simulink model "stugverter_hil"  (R2026a)
settings: Solver=VariableStepAuto  StopTime=0.8  MaxStep=1e-5
PreLoadFcn:
  | if exist('init', 'file') ~= 2,   pDir = fileparts(fileparts(which(bdroot)));   if isempty(pDir), pDir = pwd; end;   addpath(fullfile(pDir, 'scripts'));   addpath(fullfile(pDir, 'models'));   addpath(pDir); end; init;
InitFcn:
  | if exist('init', 'file') ~= 2,   pDir = fileparts(fileparts(which(bdroot)));   if isempty(pDir), pDir = pwd; end;   addpath(fullfile(pDir, 'scripts'));   addpath(fullfile(pDir, 'models'));   addpath(pDir); end; init;
undefined symbols (not defined in the file): foc, FOC_20kHz, g_duty_u, g_duty_v, g_duty_w, g_foc_exec_time_us, g_foc_isr_counter, g_hil_adc_curr_u, g_hil_adc_curr_v, g_hil_adc_curr_w, g_hil_adc_res_cos, g_hil_adc_res_sin, g_hil_mode_enable, g_spd_ref_rpm, sensor
libraries: xcpprotocollib x3
settings Model: Creator=niklasprobst  LastModifiedBy=probst
settings DebuggingCC: ParameterPrecisionLossMsg=none

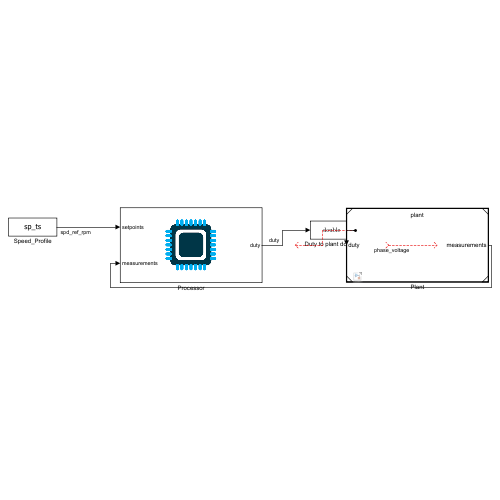
[thumbnail: Simulink's stored preview of the top-level diagram]
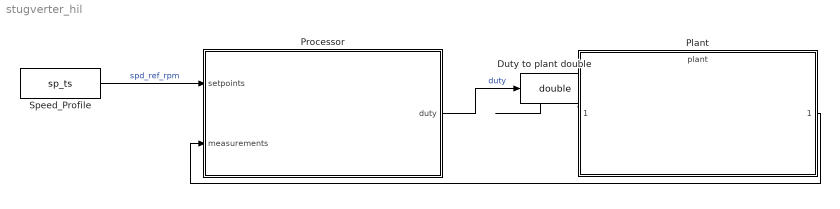
== system stugverter_hil ==
  Duty to plant double : DataTypeConversion  OutDataTypeStr=double  SaturateOnIntegerOverflow=off  RndMeth=Floor
  Plant : ModelReference  ModelNameDialog=plant  SimulationMode=Normal  ModelReferenceVersion=1.2
  Processor : Subsystem
      settings: OpenFcn=open_system(gcb, 'force');
  Speed_Profile : FromWorkspace  VariableName=sp_ts
  wires:
  Speed_Profile/1 -> Processor/1(setpoints)  "spd_ref_rpm"
  ? -> ?  "phase_voltage"
  Processor/1(duty) -> Duty to plant double/1  "duty"
  Duty to plant double/1 -> Plant/1
  Plant/1 -> Processor/2(measurements)

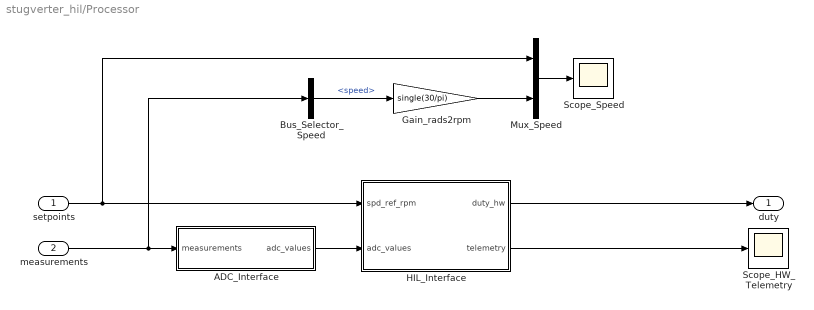
== system stugverter_hil/Processor ==
  setpoints : Inport  OutDataTypeStr=single
  measurements : Inport  Port=2  OutDataTypeStr=Bus: plant_measurement
  ADC_Interface : Subsystem
  Bus_Selector_Speed : BusSelector  OutputSignals=speed
  Gain_rads2rpm : Gain  Gain=single(30/pi)  OutDataTypeStr=single
  HIL_Interface : Subsystem
  Mux_Speed : Mux  Inputs=2
  Scope_HW_Telemetry : Scope
      settings: ActiveDisplayYMinimum=2.3463782313488107E+7  ActiveDisplayYMaximum=2.348257899228869E+7  DataLoggingVariableName=scope_hw_telemetry
  Scope_Speed : Scope
      settings: ActiveDisplayYMinimum=-579.96374511718739  ActiveDisplayYMaximum=5219.6737060546875  DataLoggingVariableName=scope_speed
  duty : Outport
  wires:
  measurements/1 -> ADC_Interface/1(measurements), Bus_Selector_Speed/1
  setpoints/1 -> HIL_Interface/1(spd_ref_rpm), Mux_Speed/1
  ADC_Interface/1(adc_values) -> HIL_Interface/2(adc_values)
  HIL_Interface/1(duty_hw) -> duty/1
  HIL_Interface/2(telemetry) -> Scope_HW_Telemetry/1
  Bus_Selector_Speed/1 -> Gain_rads2rpm/1  "<speed>"
  Gain_rads2rpm/1 -> Mux_Speed/2
  Mux_Speed/1 -> Scope_Speed/1

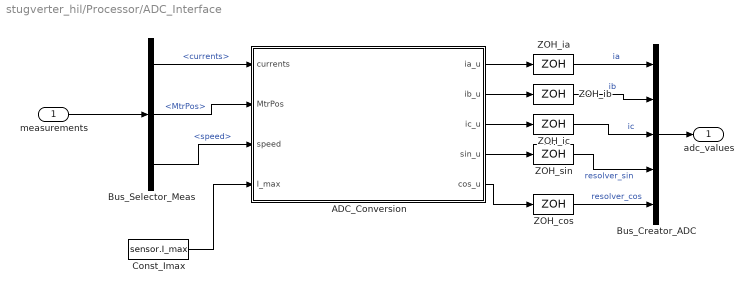
== system stugverter_hil/Processor/ADC_Interface ==
  measurements : Inport  OutDataTypeStr=Bus: plant_measurement
  ADC_Conversion : MATLAB Function  TreatAsAtomicUnit=on
  Bus_Creator_ADC : BusCreator  Inputs=5  OutDataTypeStr=Bus: adc_values  NonVirtualBus=on
  Bus_Selector_Meas : BusSelector  OutputSignals=currents,MtrPos,speed
  Const_Imax : Constant  Value=sensor.I_max
  ZOH_cos : ZeroOrderHold  SampleTime=foc.Ts
  ZOH_ia : ZeroOrderHold  SampleTime=foc.Ts
  ZOH_ib : ZeroOrderHold  SampleTime=foc.Ts
  ZOH_ic : ZeroOrderHold  SampleTime=foc.Ts
  ZOH_sin : ZeroOrderHold  SampleTime=foc.Ts
  adc_values : Outport  OutDataTypeStr=Bus: adc_values
  wires:
  measurements/1 -> Bus_Selector_Meas/1
  Bus_Selector_Meas/1 -> ADC_Conversion/1(currents)  "<currents>"
  Bus_Selector_Meas/2 -> ADC_Conversion/2(MtrPos)  "<MtrPos>"
  ADC_Conversion/1(ia_u) -> ZOH_ia/1
  ZOH_ia/1 -> Bus_Creator_ADC/1  "ia"
  ADC_Conversion/2(ib_u) -> ZOH_ib/1
  ZOH_ib/1 -> Bus_Creator_ADC/2  "ib"
  ADC_Conversion/3(ic_u) -> ZOH_ic/1
  ZOH_ic/1 -> Bus_Creator_ADC/3  "ic"
  ADC_Conversion/4(sin_u) -> ZOH_sin/1
  ZOH_sin/1 -> Bus_Creator_ADC/4  "resolver_sin"
  ADC_Conversion/5(cos_u) -> ZOH_cos/1
  ZOH_cos/1 -> Bus_Creator_ADC/5  "resolver_cos"
  Bus_Creator_ADC/1 -> adc_values/1
  Bus_Selector_Meas/3 -> ADC_Conversion/3(speed)  "<speed>"
  Const_Imax/1 -> ADC_Conversion/4(I_max)

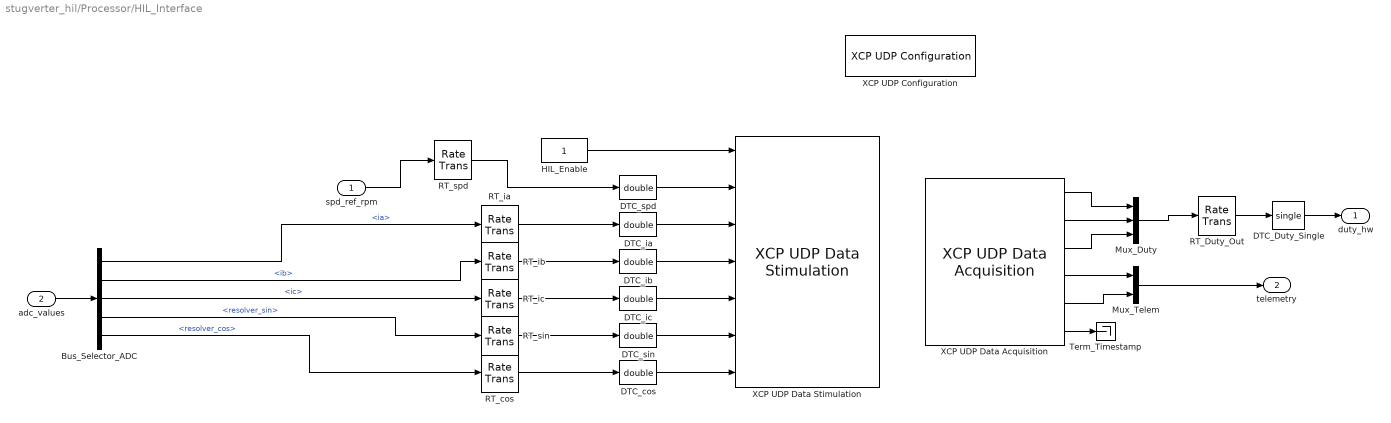
== system stugverter_hil/Processor/HIL_Interface ==
  spd_ref_rpm : Inport
  adc_values : Inport  Port=2
  Bus_Selector_ADC : BusSelector  OutputSignals=ia,ib,ic,resolver_sin,resolver_cos
  DTC_Duty_Single : DataTypeConversion  OutDataTypeStr=single  SaturateOnIntegerOverflow=off  RndMeth=Floor
  DTC_cos : DataTypeConversion  OutDataTypeStr=double  SaturateOnIntegerOverflow=off  RndMeth=Floor
  DTC_ia : DataTypeConversion  OutDataTypeStr=double  SaturateOnIntegerOverflow=off  RndMeth=Floor
  DTC_ib : DataTypeConversion  OutDataTypeStr=double  SaturateOnIntegerOverflow=off  RndMeth=Floor
  DTC_ic : DataTypeConversion  OutDataTypeStr=double  SaturateOnIntegerOverflow=off  RndMeth=Floor
  DTC_sin : DataTypeConversion  OutDataTypeStr=double  SaturateOnIntegerOverflow=off  RndMeth=Floor
  DTC_spd : DataTypeConversion  OutDataTypeStr=double  SaturateOnIntegerOverflow=off  RndMeth=Floor
  HIL_Enable : Constant  OutDataTypeStr=double  SampleTime=foc.Ts
  Mux_Duty : Mux  Inputs=3
  Mux_Telem : Mux  Inputs=2
  RT_Duty_Out : RateTransition  Deterministic=off  InitialCondition=0.5  OutPortSampleTime=foc.Ts
  RT_cos : RateTransition  Deterministic=off  InitialCondition=2048  OutPortSampleTime=foc.Ts
  RT_ia : RateTransition  Deterministic=off  InitialCondition=2048  OutPortSampleTime=foc.Ts
  RT_ib : RateTransition  Deterministic=off  InitialCondition=2048  OutPortSampleTime=foc.Ts
  RT_ic : RateTransition  Deterministic=off  InitialCondition=2048  OutPortSampleTime=foc.Ts
  RT_sin : RateTransition  Deterministic=off  InitialCondition=2048  OutPortSampleTime=foc.Ts
  RT_spd : RateTransition  Deterministic=off  OutPortSampleTime=foc.Ts
  Term_Timestamp : Terminator
  XCP UDP Configuration : xcpprotocollib/UDP/XCP UDP Configuration  Priority=-100  SlaveName=TC387  SlaveID=1  A2LFile=C:\Users\probst\Desktop\stugverter\firmware\stugverter.a2l  EnableSecurity=off  ConnectMode=off  EnableStatus=off  SampleTime=foc.Ts  HeaderErrDet=on  CTRScheme=One counter for all CTOs and DTOs  LocalAddress=192.168.0.100  LocalPort=auto  DAQTimeout=Inf
      settings: LibrarySourceBlock=vntxcplib/UDP/XCP UDP Configuration
  XCP UDP Data Acquisition : xcpprotocollib/UDP/XCP UDP Data Acquisition  SlaveName=TC387  A2LFile=C:\Users\probst\Desktop\stugverter\firmware\stugverter.a2l  EventName=FOC_20kHz (50us)  SelectedMeasurements=g_duty_u;g_duty_v;g_duty_w;g_foc_isr_counter;g_foc_exec_time_us  DAQPriority=0  SampleTime=foc.Ts  EnableTimestamp=on  InputOrOutputDatatype=Raw values as double (no Compu method conversion)
      settings: LibrarySourceBlock=vntxcplib/UDP/XCP UDP Data Acquisition
  XCP UDP Data Stimulation : xcpprotocollib/UDP/XCP UDP Data Stimulation  SlaveName=TC387  A2LFile=C:\Users\probst\Desktop\stugverter\firmware\stugverter.a2l  EventName=FOC_20kHz (50us)  SelectedMeasurements=g_hil_mode_enable;g_spd_ref_rpm;g_hil_adc_curr_u;g_hil_adc_curr_v;g_hil_adc_curr_w;g_hil_adc_res_sin;g_hil_adc_res_cos  EnableTimestamp=off  InputOrOutputDatatype=Raw values as double (no Compu method conversion)
      settings: LibrarySourceBlock=vntxcplib/UDP/XCP UDP Data Stimulation
  duty_hw : Outport
  telemetry : Outport  Port=2
  wires:
  adc_values/1 -> Bus_Selector_ADC/1
  HIL_Enable/1 -> XCP UDP Data Stimulation/1
  DTC_spd/1 -> XCP UDP Data Stimulation/2
  DTC_ia/1 -> XCP UDP Data Stimulation/3
  DTC_ib/1 -> XCP UDP Data Stimulation/4
  DTC_ic/1 -> XCP UDP Data Stimulation/5
  DTC_sin/1 -> XCP UDP Data Stimulation/6
  DTC_cos/1 -> XCP UDP Data Stimulation/7
  XCP UDP Data Acquisition/1 -> Mux_Duty/1
  XCP UDP Data Acquisition/2 -> Mux_Duty/2
  XCP UDP Data Acquisition/3 -> Mux_Duty/3
  DTC_Duty_Single/1 -> duty_hw/1
  XCP UDP Data Acquisition/4 -> Mux_Telem/1
  XCP UDP Data Acquisition/5 -> Mux_Telem/2
  Mux_Telem/1 -> telemetry/1
  XCP UDP Data Acquisition/6 -> Term_Timestamp/1
  Mux_Duty/1 -> RT_Duty_Out/1
  RT_Duty_Out/1 -> DTC_Duty_Single/1
  Bus_Selector_ADC/1 -> RT_ia/1  "<ia>"
  RT_ia/1 -> DTC_ia/1
  Bus_Selector_ADC/2 -> RT_ib/1  "<ib>"
  RT_ib/1 -> DTC_ib/1
  Bus_Selector_ADC/3 -> RT_ic/1  "<ic>"
  RT_ic/1 -> DTC_ic/1
  Bus_Selector_ADC/4 -> RT_sin/1  "<resolver_sin>"
  RT_sin/1 -> DTC_sin/1
  Bus_Selector_ADC/5 -> RT_cos/1  "<resolver_cos>"
  RT_cos/1 -> DTC_cos/1
  spd_ref_rpm/1 -> RT_spd/1
  RT_spd/1 -> DTC_spd/1

== matlab function stugverter_hil/Processor/ADC_Interface/ADC_Conversion ==
  settings: updateMethod=DISCRETE  sampleTime=foc.Ts
  data: currents input; ia_u output; MtrPos input; speed input; I_max input; ib_u output; ic_u output; sin_u output; cos_u output
function [ia_u, ib_u, ic_u, sin_u, cos_u] = fcn(currents, MtrPos, speed, I_max)
% Infineon AURIX TC387 12-bit EVADC (0..4095, midpoint 2048)
scale_I = 2047 / I_max;
ia_c = round(2048 + currents(1) * scale_I);
ib_c = round(2048 + currents(2) * scale_I);
ic_c = round(2048 + currents(3) * scale_I);
ia_u = uint16(max(0, min(4095, ia_c)));
ib_u = uint16(max(0, min(4095, ib_c)));
ic_u = uint16(max(0, min(4095, ic_c)));

% 1.5-sample PWM + transport delay compensation
pos_comp = MtrPos + 1.5 * speed * 0.00005;
sin_c = round(2048 + sin(pos_comp) * 2047);
cos_c = round(2048 + cos(pos_comp) * 2047);
sin_u = uint16(max(0, min(4095, sin_c)));
cos_u = uint16(max(0, min(4095, cos_c)));
